simulink model "Identyfikacja"  (R2015a)
settings: Solver=ode4  StartTime=0.0  StopTime=tSim  FixedStep=0.01  RelTol=1e-3
values from neighbouring files (symbols this model uses):
  c1 = Parametry(1)    [skryptDoIdentyfikacji.m]    (also in wskaznikJakosci.m = params(1))
  c2 = Parametry(2)    [skryptDoIdentyfikacji.m]    (also in wskaznikJakosci.m = params(2))
  c3 = Parametry(3)    [skryptDoIdentyfikacji.m]    (also in wskaznikJakosci.m = params(3))
settings Model: Creator=Kamil  LastModifiedBy=Kamil

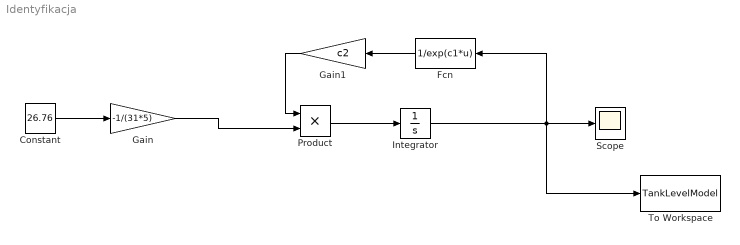
== system Identyfikacja ==
  Constant : Constant  Value=26.76
  Fcn : Fcn  Expr=1/exp(c1*u)
  Gain : Gain  Gain=-1/(31*5)
  Gain1 : Gain  Gain=c2
  Integrator : Integrator  InitialCondition=c3
  Product : Product
  Scope : Scope
      settings: TimeRange=180
  To Workspace : ToWorkspace  VariableName=TankLevelModel  SaveFormat=Structure With Time  SampleTime=-1
  wires:
  Integrator/1 -> Scope/1, To Workspace/1, Fcn/1
  Constant/1 -> Gain/1
  Gain/1 -> Product/2
  Product/1 -> Integrator/1
  Fcn/1 -> Gain1/1
  Gain1/1 -> Product/1
